simulink model "UTSG1"  (R2016a)
settings: Solver=VariableStepAuto  StartTime=0.0  StopTime=10.0  RelTol=1e-3
values from neighbouring files (symbols this model uses):
  A_dw = 110.74    [zmienne.m]
  A_fs = 60.67    [zmienne.m]
  A_p = (PI * (D_i^2) * N) / (4 * 144)    (= 11.0984259136)    [zmienne.m]
  C_1 = 1 / sqrt(C_d)    [zmienne.m]
  C_m = 0.11    [zmienne.m]
  C_p1 = 1.39    [zmienne.m]
  C_p2 = 1.165    [zmienne.m]
  DENS_d = 50.32    [zmienne.m]
  DENS_dw = 47.66    [zmienne.m]
  DENS_s = 52.32    [zmienne.m]
  DENS_w = 45.710    (= 45.71)    [zmienne.m]
  G_1 = 65.2    [zmienne.m]
  G_2 = 1.0    (= 1)    [zmienne.m]
  G_v = 32.2    [zmienne.m]
  K1 = 3.5 * 10^-6    (= 3.5e-06)    [zmienne.m]
  K2 = -7.135 * 10^-4    (= -0.0007135)    [zmienne.m]
  K3 = 0.17    [zmienne.m]
  K4 = -0.2    [zmienne.m]
  K5 = 0.14    [zmienne.m]
  K7 = 2.37 * 10^-3    (= 0.00237)    [zmienne.m]
  L = 35.54    [zmienne.m]
  L_d = 35.54    [zmienne.m]
  L_dw0 = 9.63    [zmienne.m]
  L_r = 9.63    [zmienne.m]
  m0 = 0    [zmienne.m]
  M_d = DENS_d * A_d *L_d    (= 57227.9296)    [zmienne.m]
  M_m1 = (M_m * L_s10) / L    (= 5577.64460636)    [zmienne.m]
  M_m2 = M_m * (L_s20 / L)    (= 51851.8797758)    [zmienne.m]
  M_m3 = M_m2    (= 51851.8797758)    [zmienne.m]
  M_m4 = M_m1    (= 5577.64460636)    [zmienne.m]
  M_p1 = (M_p * L_s10) / L    (= 1751.07864275)    [zmienne.m]
  M_p2 = (M_p * L_s20) / L    (= 16278.6849414)    [zmienne.m]
  P_r2 = S_pm2 / L_s20    (= 687.386379167)    [zmienne.m]
  r0 = 0    [zmienne.m]
  S_ms1 = S_m * (L_s10 / L)    (= 2678.800154)    [zmienne.m]
  S_ms2 = S_m * (L_s20 / L)    (= 24903.1326539)    [zmienne.m]
  S_ms3 = S_ms2    (= 24903.1326539)    [zmienne.m]
  S_ms4 = S_ms1    (= 2678.800154)    [zmienne.m]
  S_pm1 = (S_ms1 * D_i) / D_o    (= 2372.65156497)    [zmienne.m]
  S_pm2 = (S_ms2 * D_i) / D_o    (= 22057.0603506)    [zmienne.m]
  S_pm3 = S_pm1    (= 2372.65156497)    [zmienne.m]
  S_pm4 = S_pm2    (= 22057.0603506)    [zmienne.m]
  tau = 5    [zmienne.m]
  tau_1 = 250    [zmienne.m]
  tau_2 = 120    [zmienne.m]
  tau_pi = M_pi / W_pi    (= 0.60183806901)    [zmienne.m]
  U_ms1 = 1 / (((1 / h_os) + (D_o * log(D_o/D_m))) / (24 * K_th))    [zmienne.m]
  U_ms2 = 1 / (((1 / h_ob) + (D_o * log(D_o/D_m))) / (24 * K_th))    [zmienne.m]
  U_pm = 1 / (((1 / h_i) + (D_i * log(D_m/D_i))) / (24 * K_th))    [zmienne.m]
  V_dr = 4398.706    [zmienne.m]
  V_r = 468.981    [zmienne.m]
  w0 = 0    [zmienne.m]
  W_fi0 = 1036.39    [zmienne.m]
  W_nv = 0.63    [zmienne.m]
  W_pi = 10941.6    [zmienne.m]
  X1 = 402.94    [zmienne.m]
  X2 = 0.018    [zmienne.m]
  X3 = 1.13096    [zmienne.m]
  X4 = 370.751    [zmienne.m]
  X5 = 850.04    [zmienne.m]
  X6 = -0.181289    [zmienne.m]
  Z_tv = 3.18    [zmienne.m]
undefined symbols (not defined in the file or in its folder): magnitude
(part 2 of 2)

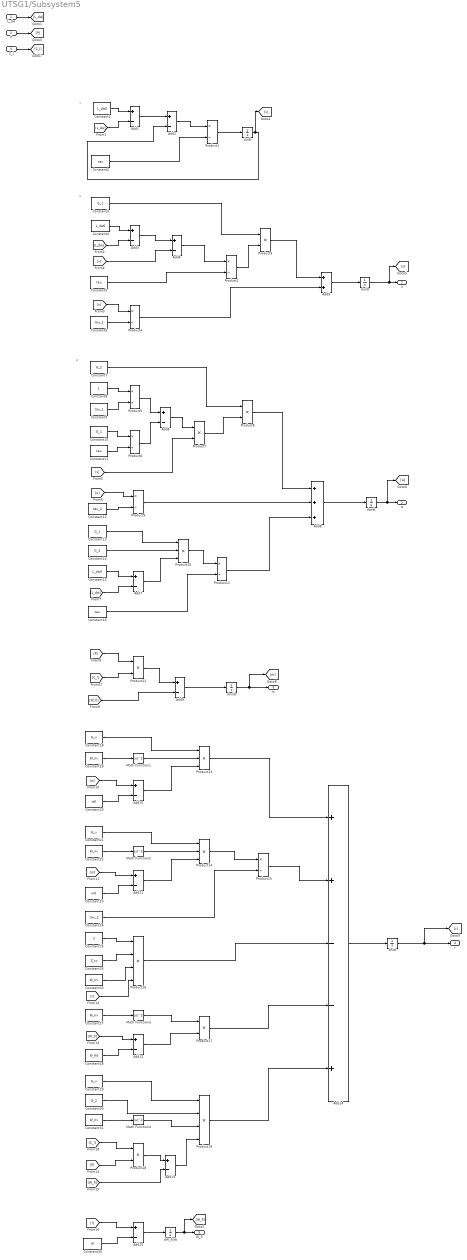
== system UTSG1/Subsystem5 ==
  note: w
  note: u
  note: v
  L_dw : Inport
  P : Inport  Port=2
  C_l : Inport  Port=3
  Add{1..4,6..7,9..13,15} (12 alike) : Sum  Inputs=+-
  Add14 : Sum  Inputs=++--+
  Add5 : Sum
  Add8 : Sum  Inputs=3
  Constant1 : Constant  Value=L_dw0
  Constant10 : Constant  Value=G_1
  Constant{2,5,11,16} (4 alike) : Constant  Value=tau
  Constant12 : Constant  Value=tau_2
  Constant13 : Constant  Value=G_1
  Constant14 : Constant  Value=G_2
  Constant15 : Constant  Value=L_dw0
  Constant18 : Constant  Value=G_v
  Constant{19,22,27,31,33} (5 alike) : Constant  Value=W_nv
  Constant20 : Constant  Value=w0
  Constant21 : Constant  Value=G_v
  Constant23 : Constant  Value=m0
  Constant24 : Constant  Value=tau_2
  Constant25 : Constant  Value=2
  Constant26 : Constant  Value=Z_tv
  Constant28 : Constant  Value=W_fi0
  Constant29 : Constant  Value=G_v
  Constant3 : Constant  Value=G_1
  Constant30 : Constant  Value=G_2
  Constant34 : Constant  Value=r0
  Constant4 : Constant  Value=L_dw0
  Constant6 : Constant  Value=tau_1
  Constant7 : Constant  Value=G_2
  Constant8 : Constant
  Constant9 : Constant  Value=tau_1
  Math Function{1..4} (4 alike) : Math  Operator=magnitude^2  SaturateOnIntegerOverflow=on
  Product{1..2,4..6,9,11,15} (8 alike) : Product  Inputs=*/
  Product10 : Product  Inputs=3
  Product{7..8,12,17..18} (5 alike) : Product
  Product13 : Product  Inputs=3
  Product14 : Product  Inputs=3
  Product16 : Product  Inputs=4
  Product19 : Product  Inputs=4
  Product3 : Product  Inputs=**
  dW_fi/dt : Integrator  InitialCondition=10941.6
  dm/dt : Integrator
  dr/dt : Integrator
  du/dt : Integrator
  dv/dt : Integrator
  dw/dt : Integrator
  u : Outport
  w : Outport  Port=2
  m : Outport  Port=3
  r : Outport  Port=4
  W_fi : Outport  Port=5
  wires:
  L_dw/1 -> [L_dw]
  P/1 -> [P]
  Constant1/1 -> Add1/1
  [L_dw] -> Add1/2
  Add1/1 -> Add2/1
  dv/dt/1 -> [v], Add2/2
  Add2/1 -> Product1/1
  Constant2/1 -> Product1/2
  Product1/1 -> dv/dt/1
  Constant4/1 -> Add3/1
  [L_dw] -> Add3/2
  Add3/1 -> Add4/1
  [v] -> Add4/2
  Add4/1 -> Product2/1
  Constant5/1 -> Product2/2
  Constant3/1 -> Product3/1
  Product2/1 -> Product3/2
  Constant6/1 -> Product4/2
  [v] -> Product4/1
  Product3/1 -> Add5/1
  Product4/1 -> Add5/2
  Add5/1 -> du/dt/1
  du/dt/1 -> [u], u/1
  Constant8/1 -> Product5/1
  Constant9/1 -> Product5/2
  Constant10/1 -> Product6/1
  Constant11/1 -> Product6/2
  Product5/1 -> Add6/1
  Product6/1 -> Add6/2
  Add6/1 -> Product7/1
  [v] -> Product7/2
  Constant7/1 -> Product8/1
  Product7/1 -> Product8/2
  [u] -> Product9/1
  Constant12/1 -> Product9/2
  Constant15/1 -> Add7/1
  [L_dw] -> Add7/2
  Constant13/1 -> Product10/1
  Constant14/1 -> Product10/2
  Add7/1 -> Product10/3
  Product10/1 -> Product11/1
  Constant16/1 -> Product11/2
  Product9/1 -> Add8/2
  Product8/1 -> Add8/1
  Product11/1 -> Add8/3
  Add8/1 -> dw/dt/1
  dw/dt/1 -> [w], w/1
  [P] -> Product12/1
  [C_l] -> Product12/2
  Product12/1 -> Add9/1
  [W_fi] -> Add9/2
  Add9/1 -> dm/dt/1
  dm/dt/1 -> [m], m/1
  Constant19/1 -> Math Function1/1
  Constant22/1 -> Math Function2/1
  Constant27/1 -> Math Function3/1
  Constant31/1 -> Math Function4/1
  [w] -> Add10/1
  Constant20/1 -> Add10/2
  [m] -> Add11/1
  Constant23/1 -> Add11/2
  [W_fi] -> Add12/1
  Constant28/1 -> Add12/2
  Constant18/1 -> Product13/1
  Math Function1/1 -> Product13/2
  Add10/1 -> Product13/3
  Constant21/1 -> Product14/1
  Math Function2/1 -> Product14/2
  Add11/1 -> Product14/3
  Product14/1 -> Product15/1
  Constant24/1 -> Product15/2
  Constant25/1 -> Product16/1
  Constant26/1 -> Product16/2
  Constant33/1 -> Product16/3
  [r] -> Product16/4
  Math Function3/1 -> Product17/1
  Add12/1 -> Product17/2
  [C_l] -> Product18/1
  [P] -> Product18/2
  Product18/1 -> Add13/1
  [W_fi] -> Add13/2
  Constant29/1 -> Product19/1
  Constant30/1 -> Product19/2
  Math Function4/1 -> Product19/3
  Add13/1 -> Product19/4
  Product13/1 -> Add14/1
  Product15/1 -> Add14/2
  Product16/1 -> Add14/3
  Product17/1 -> Add14/4
  Product19/1 -> Add14/5
  Add14/1 -> dr/dt/1
  dr/dt/1 -> [r], r/1
  [r] -> Add15/1
  Constant34/1 -> Add15/2
  Add15/1 -> dW_fi/dt/1
  dW_fi/dt/1 -> [W_fi], W_fi/1
  C_l/1 -> [C_l]
